simulink model "EvBoltCalib_Lat_v1_comb"  (R2022b)
settings: configuration reference "ConfigSetDesktopFixedStep" (kept outside this file)
PreLoadFcn:
  | VSS_BICYCLE=Simulink.Variant('Dual=0');
  | VSS_DUAL=Simulink.Variant('Dual=1');
  | Dual=1;
undefined symbols (not defined in the file or in its folder): BattChargeLimitMaxPwr, BattChargeLimitSocBpts, BattChargeLimitTbl, BattChrgCapcty, BattDischargeLimitSocBpts, BattDischargeLimitTbl, BattDischargeMaxPwr, BattNumCellsParallel, BattNumCellsSeries, BattOpenVoltCapBpts, BattOpenVoltTbl, BattResistSocBpts, BattResistTbl, BattResistTempBpts, BrakeMaxPrs, BrakeMaxTrq, ChassisDistCg2FrontAxle, ChassisDistCg2RearAxle, ChassisVehMass, DiffRatio, EnvGravCnst, EnvPrs, EnvTemp, ExpRefStructs, FuelSpecificGrav, h, InitStates, MtrEffSpdBpts, MtrEffTbl, MtrEffTrqBpts, MtrPwrMax, MtrTrqMax, SupvsryCtrlRegenBrkCutOffTbl, SupvsryCtrlRegenSpdBpts, TestScnrioCycleNum, VEH
libraries: vehdynlibtire x8, vehdynlibsuspension x7, autolibshared x6, simulink x6, autolibutils x5, VsrLibWheel x4, vehdynlibtirecommon x3, sharedtransform x3, autolibbatterycommon x2, autolibpowerinfoutils x2, autolibsharedcoupling x2, LibPtSupervisoryCtrl x2
(part 2 of 9)

== system EvBoltCalib_Lat_v1_comb/Driver/Vehicle Dynamics Blockset Complete Driver/Complete Driver ==
  TestScnrio : Inport
  Env : Inport  Port=2
  Veh : Inport  Port=3
  Bus Selector1 : BusSelector  OutputSignals=VehRefSpdLookAhead,LatRef.LatCoGDisp,GradeLookAhead
  Bus Selector2 : BusSelector  OutputSignals=Chassis.xdot,Chassis.Y,Chassis.ydot,Chassis.psi,Chassis.r
  Constant : Constant
  Constant1 : Constant
  Constant2 : Constant  Value=0
  Dead Zone : DeadZone  LowerValue=-1e-2  UpperValue=1e-2  ZeroCross=off
  Dead Zone1 : DeadZone  ZeroCross=off
  Gain : Gain  Gain=20*pi/180*18
  Predictive Driver : vehdynlibdriver/Predictive Driver  extAccelOvr=off  extDecelOvr=off  extAccelHld=off  extDecelHld=off  extAccelZero=off  extDecelZero=off  extSteerOvr=off  extSteerHld=off  extSteerZero=off  cntrlType=PI  cntrlTypeLat=Predictive  shftType=None  coordMode=SAE J670 (Z-down)  refType=Reference pose  velUnits=m/s  angUnits=rad  gearOut=off  steerOut=off  Kp=10  Ki=5  Kff=.1  Kg=0  VehVelVec=[0 100]  KffVec=[.1 .1]  KpVec=[5 5]  KiVec=[5 5]  KgVec=[0 0]  vnom=5  Kaw=1  tauerr=.01  tau=0.03  L=1  Kpt=20000  aR=200  bR=2.5  cR=.5  g=9.81  vecPose=off  dynamMode=off  PositionGainF=2.5  PositionGainR=2.5  YawRateGain=.2  DelayGain=.2  enableDrift=off  BetaRef=20*pi/180  KpBeta=1  KpDrift=2  KdDrift=1  KpPsi=6  KOmega=30  tOmega=1  a=ChassisDistCg2FrontAxle  b=ChassisDistCg2RearAxle  m=ChassisVehMass  Cy_f=5000  Cy_r=7000  I=2066  Ksteer=18  theta=40*pi/180  Idl=3  Re=.3  lambda_mu=1  GearInit=0  tShift=.1  pdlVec=[0.1 0.4 0.5 0.9]  upShftTbl=[-1 12.9375 26.4375 39.9375 51.18749999999999 62.4375 72.84375 83.25;-1 16.3125 29.8125 43.3125 54.5624 65.8125 76.78125 87.75;-1 19.6875 33.1875 46.68749999999999 57.9375 69.1875 80.71875 92.25;-1 33 52.5 77.25 100.5 138.75 161.875 185]  dwnShftTbl=[-1 12.9375 26.4375 39.9375 51.18749999999999 62.4375 72.84375 83.25;-1 16.3125 29.8125 43.3125 54.5624 65.8125 76.78125 87.75;-1 19.6875 33.1875 46.68749999999999 57.9375 69.1875 80.71875 92.25;-1 33 52.5 77.25 100.5 138.75 161.875 185]  tClutch=.5  tRev=.5  tPark=120  UpGearVec="[0  1  2  3  4  5  6  7]"  DownGearVec="[1  2  3  4  5  6  7  8]"  aMode=2
  Terminator : Terminator
  Terminator6 : Terminator
  AccelCmd : Outport
  DecelCmd : Outport  Port=2
  GearCmd : Outport  Port=3
  CltchCmd : Outport  Port=4
  IgSw : Outport  Port=5
  SteerCmd : Outport  Port=6
  wires:
  Constant/1 -> IgSw/1
  Constant1/1 -> GearCmd/1
  Env/1 -> Terminator/1
  Constant2/1 -> CltchCmd/1
  Veh/1 -> Bus Selector2/1
  Predictive Driver/3 -> AccelCmd/1
  Predictive Driver/4 -> DecelCmd/1
  Predictive Driver/2 -> Dead Zone/1
  Predictive Driver/1 -> Terminator6/1
  Dead Zone/1 -> Gain/1
  Gain/1 -> SteerCmd/1
  TestScnrio/1 -> Bus Selector1/1
  Bus Selector1/1 -> Predictive Driver/1  "<VehRefSpdLookAhead>"
  Bus Selector1/2 -> Predictive Driver/2  "<LatCoGDisp>"
  Bus Selector1/3 -> Predictive Driver/3  "<GradeLookAhead>"
  Bus Selector2/1 -> Dead Zone1/1  "<xdot>"
  Dead Zone1/1 -> Predictive Driver/4
  Bus Selector2/2 -> Predictive Driver/5  "<Y>"
  Bus Selector2/3 -> Predictive Driver/6  "<ydot>"
  Bus Selector2/4 -> Predictive Driver/7  "<psi>"
  Bus Selector2/5 -> Predictive Driver/8  "<r>"

== system EvBoltCalib_Lat_v1_comb/Driver/Vehicle Dynamics Blockset Complete Driver/Subsystem3 ==
  AccelCmd : Inport
  DecelCmd : Inport  Port=2
  GearCmd : Inport  Port=3
  CltchCmd : Inport  Port=4
  IgSw : Inport  Port=5
  SteeringCmd : Inport  Port=6
  Bus Creator : BusCreator  Inputs=6
  TransPlant : Outport
  wires:
  AccelCmd/1 -> Bus Creator/1  "AccelCmd"
  DecelCmd/1 -> Bus Creator/2  "DecelCmd"
  Bus Creator/1 -> TransPlant/1  "Driver"
  GearCmd/1 -> Bus Creator/3  "GearCmd"
  CltchCmd/1 -> Bus Creator/4  "CltchCmd"
  IgSw/1 -> Bus Creator/5  "IgSw"
  SteeringCmd/1 -> Bus Creator/6  "SteeringCmd"

== system EvBoltCalib_Lat_v1_comb/Driver/Vehicle Dynamics Blockset Longitudinal Driver /Longitudinal Driver ==
  VehRefSpd : Inport
  VehRefSpdLookAhead : Inport  Port=2
  VehDistLookAhead : Inport  Port=3
  TimeLookAhead : Inport  Port=4
  VehSpd : Inport  Port=5
  VehDist : Inport  Port=6
  RoadGrade : Inport  Port=7
  GradeLookAhead : Inport  Port=8
  Add : Sum  Inputs=+-
  Constant : Constant
  Constant1 : Constant
  Constant2 : Constant  Value=0
  Longitudinal Driver : autolibshared/Longitudinal Driver  extAccelOvr=off  extDecelOvr=off  extAccelHld=off  extDecelHld=off  extAccelZero=off  extDecelZero=off  cntrlType=PI  shftType=None  velUnits=m/s  gearOut=off  Kp=5  Ki=1  Kff=.1  Kg=0  VehVelVec=[0 100]  KffVec=[.1 .1]  KpVec=[10 10]  KiVec=[5 5]  KgVec=[0 0]  m=ChassisVehMass  Kpt=3000  tau=0.5  L=3  aR=200  bR=2.5  cR=.5  g=9.81  vnom=5  Kaw=1  tauerr=.01  tauPt=2  GearInit=0  tShift=.1  pdlVec=[0.1 0.4 0.5 0.9]  upShftTbl=[-1 12.9375 26.4375 39.9375 51.18749999999999 62.4375 72.84375 83.25;-1 16.3125 29.8125 43.3125 54.5624 65.8125 76.78125 87.75;-1 19.6875 33.1875 46.68749999999999 57.9375 69.1875 80.71875 92.25;-1 33 52.5 77.25 100.5 138.75 161.875 185]  dwnShftTbl=[1 9.5625 23.0625 36.5625 47.8125 59.0625 68.90625 78.75;1 12.9375 26.4375 39.9375 51.18749999999999 62.4375 72.84375 83.25;1 16.3125 29.8125 43.3125 54.562499 65.8125 76.78125 87.75;1 19.6875 33.1875 46.68749999999999 57.9375 69.1875 80.71875 92.25]  tClutch=.5  tRev=.5  tPark=120  aMode=2  UpGearVec="[0  1  2  3  4  5  6  7]"  DownGearVec="[1  2  3  4  5  6  7  8]"
  Scope : Scope
  Terminator{,1..5} (6 alike) : Terminator
  AccelCmd : Outport
  DecelCmd : Outport  Port=2
  GearCmd : Outport  Port=3
  CltchCmd : Outport  Port=4
  IgSw : Outport  Port=5
  wires:
  VehRefSpd/1 -> Longitudinal Driver/1
  RoadGrade/1 -> Longitudinal Driver/3
  VehSpd/1 -> Longitudinal Driver/2
  Constant/1 -> IgSw/1
  Constant1/1 -> GearCmd/1
  GradeLookAhead/1 -> Terminator4/1
  VehRefSpdLookAhead/1 -> Terminator/1
  TimeLookAhead/1 -> Terminator2/1
  Longitudinal Driver/2 -> AccelCmd/1
  Longitudinal Driver/3 -> DecelCmd/1
  Constant2/1 -> CltchCmd/1
  VehDistLookAhead/1 -> Add/1, Terminator1/1
  VehDist/1 -> Add/2, Terminator3/1
  Longitudinal Driver/1 -> Terminator5/1
  Add/1 -> Scope/1

== system EvBoltCalib_Lat_v1_comb/Driver/Vehicle Dynamics Blockset Longitudinal Driver /Subsystem1 ==
  AccelCmd : Inport
  DecelCmd : Inport  Port=2
  GearCmd : Inport  Port=3
  CltchCmd : Inport  Port=4
  IgSw : Inport  Port=5
  SteeringCmd : Inport  Port=6
  Bus Creator : BusCreator  Inputs=6
  TransPlant : Outport
  wires:
  AccelCmd/1 -> Bus Creator/1  "AccelCmd"
  DecelCmd/1 -> Bus Creator/2  "DecelCmd"
  Bus Creator/1 -> TransPlant/1  "Driver"
  GearCmd/1 -> Bus Creator/3  "GearCmd"
  CltchCmd/1 -> Bus Creator/4  "CltchCmd"
  IgSw/1 -> Bus Creator/5  "IgSw"
  SteeringCmd/1 -> Bus Creator/6  "SteeringCmd"

== system EvBoltCalib_Lat_v1_comb/Driver/Vehicle Dynamics Blockset Longitudinal Driver /Subsystem2 ==
  TestScnrio : Inport
  Env : Inport  Port=2
  Veh : Inport  Port=3
  Bus Selector : BusSelector  OutputSignals=VehRefSpd,VehRefSpdLookAhead,VehDistLookAhead,VehDist,GradeLookAhead,TimeLookAhead
  Bus Selector1 : BusSelector  OutputSignals=RoadGrade
  Bus Selector2 : BusSelector  OutputSignals=Chassis.VehSpd
  VehRefSpd : Outport
  VehRefSpdLookAhead : Outport  Port=2
  VehDistLookAhead : Outport  Port=3
  TimeLookAhead : Outport  Port=4
  VehSpd : Outport  Port=5
  VehDist : Outport  Port=6
  RoadGrade : Outport  Port=7
  GradeLookAhead : Outport  Port=8
  wires:
  TestScnrio/1 -> Bus Selector/1
  Env/1 -> Bus Selector1/1
  Bus Selector1/1 -> RoadGrade/1  "<RoadGrade>"
  Veh/1 -> Bus Selector2/1
  Bus Selector2/1 -> VehSpd/1  "<VehSpd>"
  Bus Selector/1 -> VehRefSpd/1  "<VehRefSpd>"
  Bus Selector/2 -> VehRefSpdLookAhead/1  "<VehRefSpdLookAhead>"
  Bus Selector/3 -> VehDistLookAhead/1  "<VehDistLookAhead>"
  Bus Selector/4 -> VehDist/1  "<VehDist>"
  Bus Selector/5 -> GradeLookAhead/1  "<GradeLookAhead>"
  Bus Selector/6 -> TimeLookAhead/1  "<TimeLookAhead>"

== system EvBoltCalib_Lat_v1_comb/Environment/Ground Feedback/3D Engine ==
  Friction : Inport
  Ground Z Level : Inport  Port=2
  Bus Creator : BusCreator  Inputs=4
  Bus Creator2 : BusCreator  Inputs=4
  Bus Creator3 : BusCreator  Inputs=2
  Bus Selector : BusSelector  OutputSignals=HitLoc
  Data Type Conversion : DataTypeConversion  SaturateOnIntegerOverflow=off  RndMeth=Floor
  Demux : Demux
  Demux1 : Demux
  Passenger Vehicle Ray Trace Set : sim3dlib/Vehicle Terrain Sensor  Priority=1  ActorTag=SimulinkVehicle1  VehExtEn=Constant  TireRadiiExt=Constant  VehCntrLngthVal=0  TireRadiiVal=0  VehRayLngth=10  LfRayLngth=20  RfRayLngth=20  LrRayLngth=20  RrRayLngth=20  VehRayOffset=0  LfRayOffset=-1  RfRayOffset=-1  LrRayOffset=-1  RrRayOffset=-1  VehEn=on  LfEn=on  RfEn=on  LrEn=on  RrEn=on  DbgEn=off  Ts=.03  aMode=aMode
  Rate Transition : RateTransition
  Reshape10 : Reshape  OutputDimensionality=Row vector (2-D)
  Selector1 : Selector  InputPortWidth=5  IndexOptions=Index vector (dialog)  Indices=[2:5]  OutputSizes=1
  Signal Specification : SignalSpecification  Unit=m
  Signal Specification1 : SignalSpecification  Unit=1
  Terminator : Terminator
  Terminator1 : Terminator
  Terminator2 : Terminator
  Zend Select : Selector  NumberOfDimensions=2  InputPortWidth=3  IndexOptions=Select all,Index vector (dialog)  Indices=[1 3],3  OutputSizes=1,1
  Ground : Outport  VectorParamsAs1DForOutWhenUnconnected=off
  wires:
  Selector1/1 -> Rate Transition/1
  Zend Select/1 -> Reshape10/1
  Bus Selector/1 -> Zend Select/1  "<HitLoc>"
  Passenger Vehicle Ray Trace Set/2 -> Terminator1/1
  Passenger Vehicle Ray Trace Set/3 -> Terminator2/1
  Reshape10/1 -> Selector1/1
  Passenger Vehicle Ray Trace Set/1 -> Bus Selector/1
  Rate Transition/1 -> Data Type Conversion/1
  Demux/2 -> Bus Creator/2  "G_FR_z"
  Demux/1 -> Bus Creator/1  "G_FL_z"
  Demux/4 -> Bus Creator/4  "G_RR_z"
  Demux/3 -> Bus Creator/3  "G_RL_z"
  Signal Specification/1 -> Demux/1
  Signal Specification1/1 -> Demux1/1
  Demux1/1 -> Bus Creator2/1  "mu_FL"
  Bus Creator/1 -> Bus Creator3/1  "z"
  Demux1/3 -> Bus Creator2/3  "mu_RL"
  Demux1/4 -> Bus Creator2/4  "mu_RR"
  Demux1/2 -> Bus Creator2/2  "mu_FR"
  Bus Creator2/1 -> Bus Creator3/2  "mu"
  Bus Creator3/1 -> Ground/1
  Friction/1 -> Signal Specification1/1
  Data Type Conversion/1 -> Signal Specification/1
  Ground Z Level/1 -> Terminator/1

== system EvBoltCalib_Lat_v1_comb/Environment/Ground Feedback/Constant ==
  Friction : Inport
  Ground Z Level : Inport  Port=2
  Bus Creator : BusCreator  Inputs=4
  Bus Creator2 : BusCreator  Inputs=4
  Bus Creator3 : BusCreator  Inputs=2
  Demux : Demux
  Demux1 : Demux
  Signal Specification : SignalSpecification  Unit=m
  Signal Specification1 : SignalSpecification  Unit=1
  Ground : Outport  VectorParamsAs1DForOutWhenUnconnected=off
  wires:
  Ground Z Level/1 -> Signal Specification/1
  Signal Specification/1 -> Demux/1
  Demux/4 -> Bus Creator/4  "G_RR_z"
  Demux/1 -> Bus Creator/1  "G_FL_z"
  Demux/3 -> Bus Creator/3  "G_RL_z"
  Demux/2 -> Bus Creator/2  "G_FR_z"
  Bus Creator/1 -> Bus Creator3/1  "z"
  Demux1/3 -> Bus Creator2/3  "mu_RL"
  Demux1/4 -> Bus Creator2/4  "mu_RR"
  Demux1/1 -> Bus Creator2/1  "mu_FL"
  Demux1/2 -> Bus Creator2/2  "mu_FR"
  Bus Creator2/1 -> Bus Creator3/2  "mu"
  Friction/1 -> Signal Specification1/1
  Signal Specification1/1 -> Demux1/1
  Bus Creator3/1 -> Ground/1

== system EvBoltCalib_Lat_v1_comb/Test Scenario/Drive Cycle Source/Subsystem1 ==
  LatCoGDispRef : Inport  Unit=m
  SteeringRef : Inport  Port=2  Unit=rad
  Bus Creator : BusCreator  Inputs=2
  LatRef : Outport
  wires:
  LatCoGDispRef/1 -> Bus Creator/1  "LatCoGDisp"
  Bus Creator/1 -> LatRef/1  "LatRef"
  SteeringRef/1 -> Bus Creator/2  "Steering"

== system EvBoltCalib_Lat_v1_comb/Vehicle/Battery/Battery ==
  note: Thermal model is needed to estimated battery temperature. Ambient temperture is assumed.
  Bus Creator1 : BusCreator  Inputs=1
  Bus Selector : BusSelector  OutputSignals=BattSoc
  Bus Selector2 : BusSelector  OutputSignals=Curr
  Constant : Constant  Value=EnvTemp
  Lithium Ion Battery Pack1 : Subsystem  AncestorBlock=autolibdatasheetbattery/Datasheet Battery  mask(Datasheet Battery){CapacityCtrl=Parameter, OutputVlt=Unfiltered, BattChargeMax=BattChrgCapcty, Em=BattOpenVoltTbl, CapLUTBp=BattOpenVoltCapBpts, RInt=BattResistTbl, BattTempBp=BattResistTempBpts, CapSOCBp=BattResistSocBpts, Ns=BattNumCellsSeries, Np=BattNumCellsParallel, BattCapInit=InitStates(TestScnrioCycleNum).BattSoc*BattChrgCapcty, Tc=1/1000, Vinit=3.75*72, RefBlkName='autolibdatasheetbattery/Datasheet Battery'}
      mask prompts: CapacityCtrl "autoblks:autoblkDatasheetBattery:blkPrm_CapacityCtrl"; OutputVlt "autoblks:autoblkDatasheetBattery:blkPrm_OutputVlt"; BattChargeMax "autoblks:autoblkDatasheetBattery:blkPrm_BattChargeMax"; Em "autoblks:autoblkDatasheetBattery:blkPrm_Em"; CapLUTBp "autoblks:autoblkDatasheetBattery:blkPrm_CapLUTBp"; RInt "autoblks:autoblkDatasheetBattery:blkPrm_RInt"; BattTempBp "autoblks:autoblkDatasheetBattery:blkPrm_BattTempBp"; CapSOCBp "autoblks:autoblkDatasheetBattery:blkPrm_CapSOCBp"; Ns "autoblks:autoblkDatasheetBattery:blkPrm_Ns"; Np "autoblks:autoblkDatasheetBattery:blkPrm_Np"; BattCapInit "autoblks:autoblkDatasheetBattery:blkPrm_BattCapInit"; Tc "autoblks:autoblkDatasheetBattery:blkPrm_Tc"; Vinit "autoblks:autoblkDatasheetBattery:blkPrm_Vinit"
      mask help: autoblks:autoblkDatasheetBattery:blkDesc
      mask init:
      | autoicon('autolibdatasheetbattery',gcb,'Initialization');
      settings: LibrarySourceBlock=autolibdatasheetbattery/Datasheet Battery
      mask Help: eval('autoblkshelp(''pbbatterydatasheet'')');
      mask TypeOptions CapacityCtrl: autoblks:autoblkDatasheetBattery:blkCmb_CapacityCtrlExternalInput | autoblks:autoblkDatasheetBattery:blkCmb_CapacityCtrlParameter
      mask TypeOptions OutputVlt: autoblks:autoblkDatasheetBattery:blkCmb_OutputVltFiltered | autoblks:autoblkDatasheetBattery:blkCmb_OutputVltUnfiltered
      mask DialogControl Container3 Prompt: autoblks:autoblkDatasheetBattery:blkDlg_Container3
      mask DialogControl CapacityCtrl Prompt: Initial battery capacity:
      mask DialogControl OutputVlt Prompt: Output battery voltage:
      mask DialogControl ParameterGroupVar Prompt: autoblks:autoblkDatasheetBattery:blkDlg_ParameterGroupVar
      mask DialogControl BattChargeMax Prompt: Rated capacity at nominal temperature, BattChargeMax [Ah]:
      mask DialogControl Em Prompt: Open circuit voltage table data, Em [V]:
      mask DialogControl CapLUTBp Prompt: Open circuit voltage breakpoints 1, CapLUTBp []:
      mask DialogControl RInt Prompt: Internal resistance table data, RInt [Ohms]:
      mask DialogControl BattTempBp Prompt: Battery temperature breakpoints 1, BattTempBp [K]:
      mask DialogControl CapSOCBp Prompt: Battery capacity breakpoints 2, CapSOCBp []:
      mask DialogControl Ns Prompt: Number of cells in series, Ns []:
      mask DialogControl Np Prompt: Number of cells in parallel, Np []:
      mask DialogControl BattCapInit Prompt: Initial battery capacity, BattCapInit [Ah]:
      mask DialogControl Tc Prompt: Output battery voltage time constant, Tc [s]:
      mask DialogControl Vinit Prompt: Output battery voltage initial value, Vinit [V]:
      mask Display:
      | IconInfo = autoicon('autolibdatasheetbattery', gcb, 'DrawCommands');
      | 
      | image(IconInfo.image, IconInfo.position);
      | 
      | for i = 1:numel(IconInfo.lconn)
      |     port_label('lconn', i, IconInfo.lconn{i})
      | end
      | 
      | for j = 1:numel(IconInfo.rconn)
      |     port_label('rconn', j, IconInfo.rconn{j})
      | end
      | 
      | for k = 1:numel(IconInfo.input)
      |     port_label('input', k, IconInfo.input{k})
      | end
      | 
      | for m = 1:numel(IconInfo.output)
      |     port_label('output', m, IconInfo.output{m})
      | end
  Two-Way Connection1 : TwoWayConnection
  Batt : PMIOPort  Side=Right
  BattSoc : Outport
  BattCurr : Outport  Port=2  Unit=A
  BattVolt : Outport  Port=3  Unit=V
  wires:
  Bus Selector2/1 -> Lithium Ion Battery Pack1/1(BattCurr), BattCurr/1  "<Curr>"
  Lithium Ion Battery Pack1/2(BattVolt) -> BattVolt/1, Bus Creator1/1  "Volt"
  Bus Creator1/1 -> Two-Way Connection1/1
  Constant/1 -> Lithium Ion Battery Pack1/2(BattTemp)
  Bus Selector/1 -> BattSoc/1  "<BattSoc>"
  Lithium Ion Battery Pack1/1(Info) -> Bus Selector/1
  Two-Way Connection1/1 -> Bus Selector2/1
  connections:
  Batt/RConn1 -- Two-Way Connection1/RConn1

== system EvBoltCalib_Lat_v1_comb/Vehicle/Battery/Subsystem1 ==
  BattSoc : Inport
  BattCurr : Inport  Port=2
  BattVolt : Inport  Port=3
  Bus Creator : BusCreator  Inputs=3
  Batt : Outport
  wires:
  BattSoc/1 -> Bus Creator/1  "BattSoc"
  BattCurr/1 -> Bus Creator/2  "BattCurr"
  Bus Creator/1 -> Batt/1  "Batt"
  BattVolt/1 -> Bus Creator/3  "BattVolt"

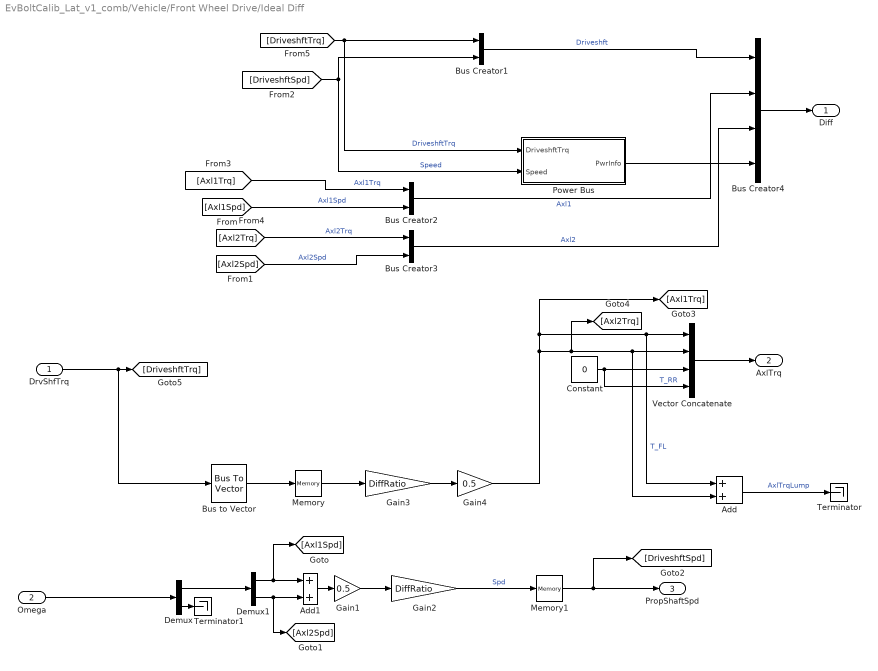
== system EvBoltCalib_Lat_v1_comb/Vehicle/Front Wheel Drive/Ideal Diff ==
  DrvShfTrq : Inport
  Omega : Inport  Port=2
  Add : Sum
  Add1 : Sum
  Bus Creator1 : BusCreator  Inputs=2
  Bus Creator2 : BusCreator  Inputs=2
  Bus Creator3 : BusCreator  Inputs=2
  Bus Creator4 : BusCreator  Inputs=4
  Bus to Vector : BusToVector
  Constant : Constant  Value=0
  Demux : Demux  Outputs=[2,2]
  Demux1 : Demux  Outputs=2
  Gain1 : Gain  Gain=0.5
  Gain2 : Gain  Gain=DiffRatio
  Gain3 : Gain  Gain=DiffRatio
  Gain4 : Gain  Gain=0.5
  Memory : Memory
  Memory1 : Memory
  Power Bus : Subsystem
  Terminator : Terminator
  Terminator1 : Terminator
  Vector Concatenate : Concatenate  NumInputs=4
  Diff : Outport  VectorParamsAs1DForOutWhenUnconnected=off
  AxlTrq : Outport  Port=2  VectorParamsAs1DForOutWhenUnconnected=off
  PropShaftSpd : Outport  Port=3  VectorParamsAs1DForOutWhenUnconnected=off
  wires:
  Demux1/2 -> [Axl2Spd], Add1/2
  Vector Concatenate/1 -> AxlTrq/1
  Gain4/1 -> [Axl1Trq], Add/1, Vector Concatenate/1, [Axl2Trq], Add/2, Vector Concatenate/2  "T_FL"
  DrvShfTrq/1 -> [DriveshftTrq], Bus to Vector/1
  [DriveshftTrq] -> Power Bus/1(DriveshftTrq), Bus Creator1/1  "DriveshftTrq"
  [Axl1Spd] -> Bus Creator2/2  "Axl1Spd"
  Demux/1 -> Demux1/1
  Add1/1 -> Gain1/1
  Bus Creator4/1 -> Diff/1
  Add/1 -> Terminator/1  "AxlTrqLump"
  [Axl2Trq] -> Bus Creator3/1  "Axl2Trq"
  Omega/1 -> Demux/1
  Memory/1 -> Gain3/1
  Bus to Vector/1 -> Memory/1
  Bus Creator3/1 -> Bus Creator4/3  "Axl2"
  Bus Creator2/1 -> Bus Creator4/2  "Axl1"
  Bus Creator1/1 -> Bus Creator4/1  "Driveshft"
  [DriveshftSpd] -> Bus Creator1/2, Power Bus/2(Speed)  "Speed"
  Gain2/1 -> Memory1/1  "Spd"
  Constant/1 -> Vector Concatenate/4, Vector Concatenate/3  "T_RR"
  Demux1/1 -> [Axl1Spd], Add1/1
  Memory1/1 -> PropShaftSpd/1, [DriveshftSpd]
  Gain3/1 -> Gain4/1
  [Axl1Trq] -> Bus Creator2/1  "Axl1Trq"
  Power Bus/1(PwrInfo) -> Bus Creator4/4
  Gain1/1 -> Gain2/1
  [Axl2Spd] -> Bus Creator3/2  "Axl2Spd"
  Demux/2 -> Terminator1/1

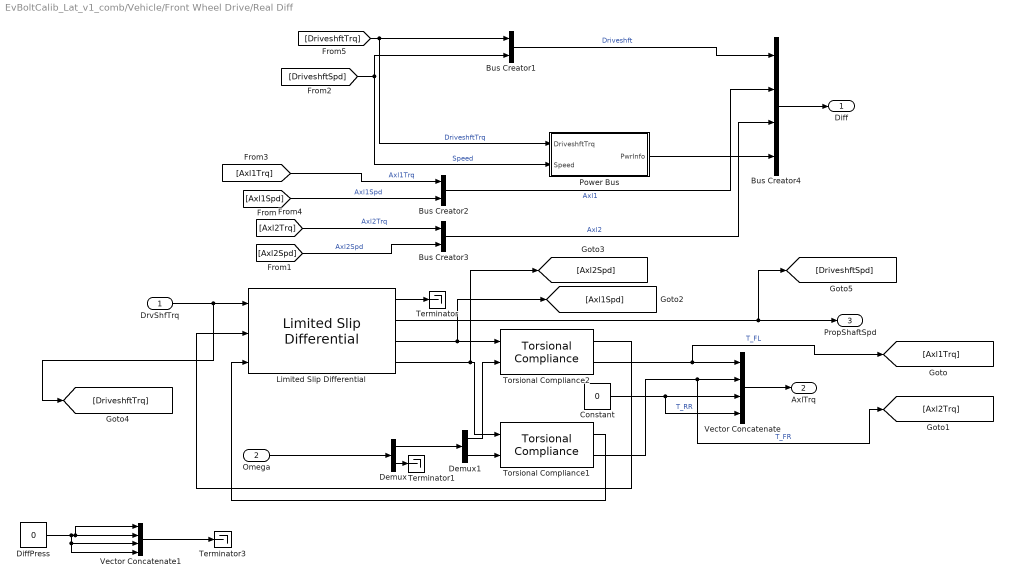
== system EvBoltCalib_Lat_v1_comb/Vehicle/Front Wheel Drive/Real Diff ==
  DrvShfTrq : Inport
  Omega : Inport  Port=2
  Bus Creator1 : BusCreator  Inputs=2
  Bus Creator2 : BusCreator  Inputs=2
  Bus Creator3 : BusCreator  Inputs=2
  Bus Creator4 : BusCreator  Inputs=4
  Constant : Constant  Value=0
  Demux : Demux  Outputs=[2,2]
  Demux1 : Demux  Outputs=2
  DiffPress : Constant  Value=0
  Limited Slip Differential : autolibshareddiff/Limited Slip Differential  DiffEffModelPopup=Constant  InterpMethod=Linear point-slope  extTamb=off  shaftSwitchMask=To the left of center-line  Ndiff=7.05  Jd=0.025  bd=1e-3  Jw1=0.01  bw1=1e-3  Jw2=0.01  bw2=1e-3  omegaw1o=0  omegaw2o=0  eta=0.98  eta_tbl=reshape([0.64 0.76 0.8 0.81 0.83 0.84 0.84 0.56 0.73 0.78 0.8 0.83 0.84 0.84 0.54 0.71 0.77 0.8 0.82 0.84 0.84 0.53 0.71 0.77 0.8 0.83 0.84 0.84 0.51 0.71 0.77 0.8 0.83 0.84 0.85 0.52 0.7 0.77 0.8 0.83 0.84 0.85 0.51 0.71 0.76 0.79 0.83 0.84 0.85 0.5 0.69 0.76 0.79 0.82 0.84 0.85 0.45 0.68 0.75 0.78 0.82 0.84 0.85 0.43 0.67 0.74 0.78 0.81 0.83 0.84 0.38 0.63 0.71 0.75 0.8 0.82 0.83 0.81 0.86 0.88 0.89 0.89 0.89 0.9 0.77 0.85 0.87 0.88 0.89 0.9 0.9 0.72 0.82 0.86 0.87 0.88 0.89 0.9 0.68 0.8 0.84 0.86 0.88 0.89 0.89 0.67 0.8 0.84 0.86 0.88 0.89 0.9 0.67 0.8 0.84 0.86 0.88 0.89 0.9 0.65 0.8 0.84 0.86 0.88 0.89 0.9 0.64 0.79 0.83 0.86 0.88 0.89 0.9 0.63 0.78 0.83 0.86 0.88 0.89 0.9 0.59 0.76 0.82 0.85 0.87 0.89 0.9 0.53 0.73 0.8 0.83 0.86 0.88 0.89], 7, 11, 2)  Trq_bpts=[25, 50, 75, 100, 150, 200, 250]  omega_bpts=[52.4 78.5 105 131 157 183 209 262 314 419 524]  Temp_bpts=[290 358]  Tamb=297.15  couplingType=Pre-loaded ideal clutch  Ndisks=8  Reff=.08  Fc=1000  muc=[.16 0.13 0.115 0.11 0.105 0.1025 0.10125 .10125]  dw=[0 10 20 40 60 80 100 1000]  Tdw=[-100, -90, -50, -5, 0, 5, 50, 90, 100]  dwT=[-200, -175, -100, - 50, 0, 50, 100, 175, 200]  TTin=[-200 -175 -100 - 50 0 50 100 175 200]  Tin=[-200 -175 -100 - 50 0 50 100 175 200]  tauC=.04  IdealInterpMethod=Linear point-slope  IdealExtrapMethod=Linear  TdwInterpMethod=Flat  TdwExtrapMethod=Clip  TTinInterpMethod=Flat  TTinExtrapMethod=Clip  maxAbsSpd=5e3  aMode=2
  Power Bus : Subsystem
  Terminator : Terminator
  Terminator1 : Terminator
  Terminator3 : Terminator
  Torsional Compliance1 : autolibsharedcoupling/Torsional Compliance  port_config=Simulink  extInfo=off  k=10000  b=400  theta_o=0  domega_o=0  omega_c=300  blkID=0  aMode=2
  Torsional Compliance2 : autolibsharedcoupling/Torsional Compliance  port_config=Simulink  extInfo=off  k=10000  b=400  theta_o=0  domega_o=0  omega_c=300  blkID=0  aMode=2
  Vector Concatenate : Concatenate  NumInputs=4
  Vector Concatenate1 : Concatenate  NumInputs=4
  Diff : Outport  VectorParamsAs1DForOutWhenUnconnected=off
  AxlTrq : Outport  Port=2  VectorParamsAs1DForOutWhenUnconnected=off
  PropShaftSpd : Outport  Port=3  VectorParamsAs1DForOutWhenUnconnected=off
  wires:
  Limited Slip Differential/3 -> [Axl1Spd], Torsional Compliance2/1
  Demux1/1 -> Torsional Compliance2/2
  Limited Slip Differential/1 -> Terminator/1
  DrvShfTrq/1 -> [DriveshftTrq], Limited Slip Differential/1
  Limited Slip Differential/4 -> [Axl2Spd], Torsional Compliance1/1
  Demux1/2 -> Torsional Compliance1/2
  Demux/1 -> Demux1/1
  Torsional Compliance1/1 -> Limited Slip Differential/3
  Torsional Compliance2/1 -> Limited Slip Differential/2
  Demux/2 -> Terminator1/1
  Constant/1 -> Vector Concatenate/4, Vector Concatenate/3  "T_RR"
  Torsional Compliance1/2 -> [Axl2Trq], Vector Concatenate/2  "T_FR"
  Torsional Compliance2/2 -> [Axl1Trq], Vector Concatenate/1  "T_FL"
  Omega/1 -> Demux/1
  Vector Concatenate/1 -> AxlTrq/1
  Vector Concatenate1/1 -> Terminator3/1
  DiffPress/1 -> Vector Concatenate1/4, Vector Concatenate1/3, Vector Concatenate1/1, Vector Concatenate1/2
  [DriveshftTrq] -> Power Bus/1(DriveshftTrq), Bus Creator1/1  "DriveshftTrq"
  [Axl1Spd] -> Bus Creator2/2  "Axl1Spd"
  [Axl2Trq] -> Bus Creator3/1  "Axl2Trq"
  Bus Creator4/1 -> Diff/1
  [Axl2Spd] -> Bus Creator3/2  "Axl2Spd"
  [DriveshftSpd] -> Bus Creator1/2, Power Bus/2(Speed)  "Speed"
  Bus Creator1/1 -> Bus Creator4/1  "Driveshft"
  [Axl1Trq] -> Bus Creator2/1  "Axl1Trq"
  Power Bus/1(PwrInfo) -> Bus Creator4/4
  Bus Creator2/1 -> Bus Creator4/2  "Axl1"
  Bus Creator3/1 -> Bus Creator4/3  "Axl2"
  Limited Slip Differential/2 -> [DriveshftSpd], PropShaftSpd/1

== system EvBoltCalib_Lat_v1_comb/Vehicle/Powertrain Supervisory Controller /Engine Torque Command ==
  AccelCmdIn : Inport
  DecelCmdIn : Inport  Port=2
  DriverGearCmdIn : Inport  Port=3
  VehSpd : Inport  Port=4
  BattSoc : Inport  Port=5
  MtrSpd : Inport  Port=6
  Accel Pedal to Traction Wheel Torque Request1 : Subsystem
  Battery Management System : Subsystem
  Motor Torque Arbitration and Power Management : Subsystem
  Series Regen Braking : Subsystem  InitFcn=%[~]=autosharedicon('autolibutils',gcb,0);  VariantControl=Variant
  MtrTrqCmd : Outport
  AccelCmd : Outport  Port=2
  BrkCmd : Outport  Port=3
  DriverGearCmd : Outport  Port=4
  wires:
  DecelCmdIn/1 -> Series Regen Braking/4("DecelCmd ")  "DecelPdl"
  DriverGearCmdIn/1 -> DriverGearCmd/1
  [AccelPdl] -> Motor Torque Arbitration and Power Management/2(AccelPdl)
  MtrSpd/1 -> [MotSpd], Series Regen Braking/3(MotSpd)  "MotSpd"
  AccelCmdIn/1 -> AccelCmd/1, Accel Pedal to Traction Wheel Torque Request1/1(AccelPdl), [AccelPdl]
  VehSpd/1 -> [VehSpd], Series Regen Braking/2(VehSpd)  "VehSpd"
  BattSoc/1 -> Battery Management System/1(SOC), Series Regen Braking/1(BattSoc)  "SOC"
  Battery Management System/1(BattPwrDischrgLmt) -> Motor Torque Arbitration and Power Management/3(BattPwrDisChrgLmt)  "BattPwrDischrgLmt"
  Series Regen Braking/2(" BrkCmd") -> BrkCmd/1  "BrkCmd"
  Battery Management System/2(BattPwrChrgLmt) -> Motor Torque Arbitration and Power Management/4("BattPwrChrgLmt ")  "BattPwrChrgLmt"
  Series Regen Braking/1(" MotTrqCmdRegen") -> Motor Torque Arbitration and Power Management/6(MotTrqCmdRegen)  "MotTrqCmdRegen"
  [MotSpd] -> Motor Torque Arbitration and Power Management/5(MotSpd)
  Motor Torque Arbitration and Power Management/1(MotTrqCmdFinal) -> MtrTrqCmd/1  "MotTrqCmd"
  [VehSpd] -> Accel Pedal to Traction Wheel Torque Request1/2(MotSpd)
  Accel Pedal to Traction Wheel Torque Request1/1(TrqCmd) -> Motor Torque Arbitration and Power Management/1(MotTrqCmdTrac)

== system EvBoltCalib_Lat_v1_comb/Vehicle/Powertrain Supervisory Controller /Subsystem1 ==
  MtrTrqCmd : Inport
  AccelCmd : Inport  Port=2
  BrkCmd : Inport  Port=3
  DriverGearCmd : Inport  Port=4
  SteeringCmd : Inport  Port=5
  Bus Creator : BusCreator  Inputs=5
  SupvsryCtrl : Outport
  wires:
  MtrTrqCmd/1 -> Bus Creator/1  "MtrTrqCmd"
  Bus Creator/1 -> SupvsryCtrl/1  "SupvsryCtrl"
  AccelCmd/1 -> Bus Creator/2  "AccelCmd"
  BrkCmd/1 -> Bus Creator/3  "BrkCmd"
  DriverGearCmd/1 -> Bus Creator/4  "DriverGearCmd"
  SteeringCmd/1 -> Bus Creator/5  "SteeringCmd"

== system EvBoltCalib_Lat_v1_comb/Vehicle/Powertrain Supervisory Controller /Subsystem4 ==
  Driver : Inport
  Chassis : Inport  Port=2
  Batt : Inport  Port=3
  Mtr : Inport  Port=4
  Bus Selector : BusSelector  OutputSignals=AccelCmd,DecelCmd,GearCmd
  Bus Selector1 : BusSelector  OutputSignals=VehSpd
  Bus Selector2 : BusSelector  OutputSignals=BattSoc
  Bus Selector3 : BusSelector  OutputSignals=MtrSpd
  AccelCmd : Outport  VectorParamsAs1DForOutWhenUnconnected=off
  DecelCmd : Outport  Port=2  VectorParamsAs1DForOutWhenUnconnected=off
  DriverGearCmd : Outport  Port=3  VectorParamsAs1DForOutWhenUnconnected=off
  VehSpd : Outport  Port=4  VectorParamsAs1DForOutWhenUnconnected=off
  BattSoc : Outport  Port=5  VectorParamsAs1DForOutWhenUnconnected=off
  MtrSpd : Outport  Port=6  VectorParamsAs1DForOutWhenUnconnected=off
  wires:
  Driver/1 -> Bus Selector/1
  Bus Selector/1 -> AccelCmd/1  "<AccelCmd>"
  Bus Selector/3 -> DriverGearCmd/1  "<GearCmd>"
  Chassis/1 -> Bus Selector1/1
  Bus Selector1/1 -> VehSpd/1  "<VehSpd>"
  Bus Selector/2 -> DecelCmd/1  "<DecelCmd>"
  Batt/1 -> Bus Selector2/1
  Bus Selector2/1 -> BattSoc/1  "<BattSoc>"
  Mtr/1 -> Bus Selector3/1
  Bus Selector3/1 -> MtrSpd/1  "<MtrSpd>"

== system EvBoltCalib_Lat_v1_comb/Vehicle/Vehicle Dynamics/Vehicle 14DOF ==
  Env : Inport
  SupvsryCtrl : Inport  Port=2
  AxlTrq : Inport  Port=3
  Brake Pressure : Subsystem
  Bus Selector : BusSelector  OutputSignals=SteeringCmd
  Bus Selector1 : BusSelector  OutputSignals=BrkCmd
  Bus Selector2 : BusSelector  OutputSignals=WindVel,GndBus.z,GndBus.mu
  Bus Selector3 : BusSelector  OutputSignals=G_FL_z,G_FR_z,G_RL_z,G_RR_z
  Bus Selector4 : BusSelector  OutputSignals=mu_FL,mu_FR,mu_RL,mu_RR
  Constant : Constant  Value=0
  Steering : Subsystem
  Subsystem4 : Subsystem
  Suspension : Subsystem  Variant=on  VariantControlMode=label  LabelModeActiveChoice=3
      mask Display:
      | switch str2num(get_param(gcb,'ActiveVariant'))
      |     case 1
      |         image('suspdw.png');
      |     case 2
      |         image([imread('suspindmap.png');imread('suspsamap.png')]);
      |     case 3
      |          image([imread('suspmacp.png');imread('suspsacoil.png')]);
      |     case 4
      |          image('suspmacp.png');
      |     case 5
      |          image('suspindmap.png');
      | end
  Vector Concatenate : Concatenate  NumInputs=4
  Vector Concatenate1 : Concatenate  NumInputs=4
  Vector Concatenate2 : Concatenate  NumInputs=4
  Vehicle : Subsystem
      mask Display: image('6dofcar.png');
  Vehicle Routing : Subsystem
  Wheel Routing : Subsystem
  Wheels and Tires : Subsystem
      mask Display: image('wheel3dof.png')
  Whl : Outport
  Chassis : Outport  Port=2
  wires:
  Vehicle Routing/9(GeomXYZdot) -> Subsystem4/9(GeomXYZdot)
  Vehicle Routing/8(GeomXYZ) -> Subsystem4/8(GeomXYZ)
  Vehicle Routing/1(Cgxyzdot) -> Subsystem4/1(Cgxyzdot)
  Vehicle Routing/5(pqr) -> Subsystem4/5(pqr)
  Vehicle Routing/4(angles) -> Subsystem4/4(angles)
  Vehicle Routing/3(CgXYZdot) -> Subsystem4/3(CgXYZdot)
  Vehicle Routing/7(Beta) -> Subsystem4/7(Beta)
  Wheels and Tires/1(Wheels) -> Wheel Routing/2(Wheel), Suspension/3(Wheel)  "Wheels"
  Vehicle Routing/2(CgXYZ) -> Subsystem4/2(CgXYZ)
  Vehicle/1(VehFdbk) -> Suspension/2(Vehicle), Wheel Routing/1(Info), Vehicle Routing/1(Veh)  "Veh"
  Suspension/1(Suspension) -> Vehicle/1(Suspension), Wheels and Tires/1(Suspension)  "Susp"
  Bus Selector2/1 -> Vehicle/2(Wind)  "<WindVel>"
  Steering/1(WhlAng) -> Suspension/1(Steering)
  Bus Selector/1 -> Steering/1(SteeringCmd)  "<SteeringCmd>"
  SupvsryCtrl/1 -> Bus Selector/1, Bus Selector1/1
  Bus Selector1/1 -> Brake Pressure/1(BrkReq)  "<BrkCmd>"
  Env/1 -> Bus Selector2/1
  Vehicle Routing/6(Cgaxyz) -> Subsystem4/6(Cgaxyz)
  Wheel Routing/1(Omega) -> Subsystem4/10(Omega)
  Wheel Routing/3(Alpha) -> Subsystem4/12(Alpha)
  Wheel Routing/4(XWheel) -> Subsystem4/13(XWheel)
  Wheel Routing/2(Kappa) -> Subsystem4/11(Kappa)
  Wheel Routing/5(YWheel) -> Subsystem4/14(YWheel)
  Wheel Routing/6(ZWheel) -> Subsystem4/15(dzWheel)
  Subsystem4/2(Wheels) -> Whl/1
  Subsystem4/1(Chassis) -> Chassis/1
  AxlTrq/1 -> Wheels and Tires/2(Axle Torque)
  Bus Selector2/2 -> Bus Selector3/1  "<z>"
  Bus Selector3/1 -> Vector Concatenate/1  "<G_FL_z>"
  Bus Selector3/2 -> Vector Concatenate/2  "<G_FR_z>"
  Bus Selector3/3 -> Vector Concatenate/3  "<G_RL_z>"
  Bus Selector3/4 -> Vector Concatenate/4  "<G_RR_z>"
  Vector Concatenate/1 -> Wheels and Tires/4(Ground Input)
  Bus Selector4/4 -> Vector Concatenate1/4  "<mu_RR>"
  Bus Selector2/3 -> Bus Selector4/1  "<mu>"
  Bus Selector4/3 -> Vector Concatenate1/3  "<mu_RL>"
  Bus Selector4/2 -> Vector Concatenate1/2  "<mu_FR>"
  Bus Selector4/1 -> Vector Concatenate1/1  "<mu_FL>"
  Vector Concatenate1/1 -> Wheels and Tires/5(Friction)
  Constant/1 -> Vector Concatenate2/4, Vector Concatenate2/3, Vector Concatenate2/2, Vector Concatenate2/1
  Brake Pressure/1(BrakePrs) -> Wheels and Tires/3(Brake Press)

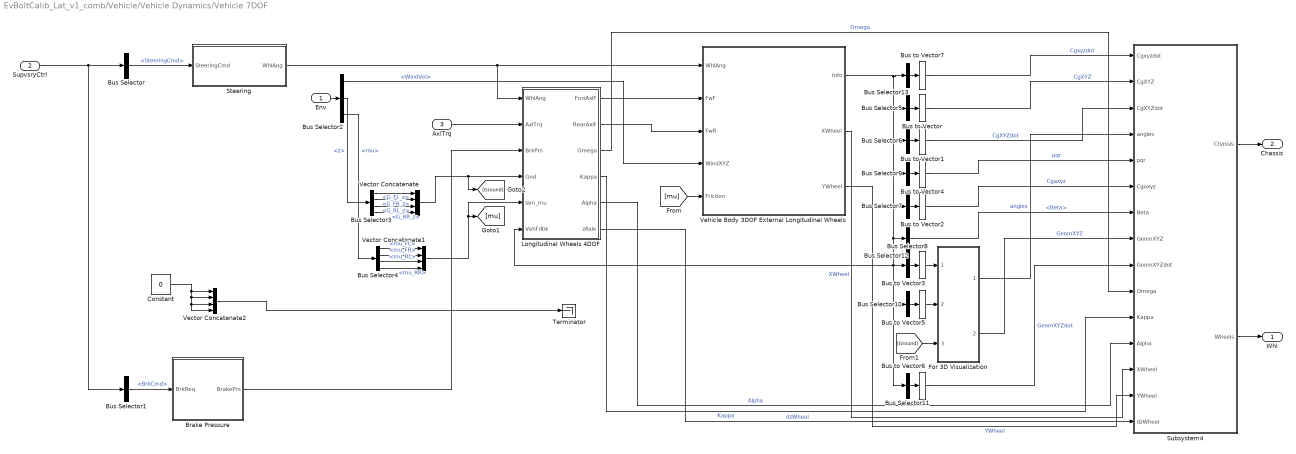
== system EvBoltCalib_Lat_v1_comb/Vehicle/Vehicle Dynamics/Vehicle 7DOF ==
  Env : Inport
  SupvsryCtrl : Inport  Port=2
  AxlTrq : Inport  Port=3
  Brake Pressure : Subsystem
  Bus Selector : BusSelector  OutputSignals=SteeringCmd
  Bus Selector1 : BusSelector  OutputSignals=BrkCmd
  Bus Selector10 : BusSelector  OutputSignals=InertFrm.Geom.Disp.X,InertFrm.Geom.Disp.Y,InertFrm.Geom.Disp.Z  OutputAsBus=on
  Bus Selector11 : BusSelector  OutputSignals=InertFrm.Geom.Vel.Xdot,InertFrm.Geom.Vel.Ydot,InertFrm.Geom.Vel.Zdot  OutputAsBus=on
  Bus Selector12 : BusSelector  OutputSignals=BdyFrm.Geom.Ang.Beta
  Bus Selector13 : BusSelector  OutputSignals=BdyFrm.Cg.Vel.xdot,BdyFrm.Cg.Vel.ydot,BdyFrm.Cg.Vel.zdot  OutputAsBus=on
  Bus Selector2 : BusSelector  OutputSignals=WindVel,GndBus.z,GndBus.mu
  Bus Selector3 : BusSelector  OutputSignals=G_FL_z,G_FR_z,G_RL_z,G_RR_z
  Bus Selector4 : BusSelector  OutputSignals=mu_FL,mu_FR,mu_RL,mu_RR
  Bus Selector5 : BusSelector  OutputSignals=InertFrm.Cg.Disp.X,InertFrm.Cg.Disp.Y,InertFrm.Cg.Disp.Z  OutputAsBus=on
  Bus Selector6 : BusSelector  OutputSignals=InertFrm.Cg.Vel.Xdot,InertFrm.Cg.Vel.Ydot,InertFrm.Cg.Vel.Zdot  OutputAsBus=on
  Bus Selector7 : BusSelector  OutputSignals=BdyFrm.Cg.Acc.ax,BdyFrm.Cg.Acc.ay,BdyFrm.Cg.Acc.az  OutputAsBus=on
  Bus Selector8 : BusSelector  OutputSignals=InertFrm.Cg.Ang.phi,InertFrm.Cg.Ang.theta,InertFrm.Cg.Ang.psi  OutputAsBus=on
  Bus Selector9 : BusSelector  OutputSignals=BdyFrm.Cg.AngVel.p,BdyFrm.Cg.AngVel.q,BdyFrm.Cg.AngVel.r  OutputAsBus=on
  Bus to Vector{,1..7} (8 alike) : BusToVector
  Constant : Constant  Value=0
  For 3D Visualization : MATLAB Function  TreatAsAtomicUnit=on  mask{trackW=1.9, wheelB=ChassisDistCg2FrontAxle+ChassisDistCg2RearAxle}
      mask prompts: trackW "Vehicle track width, trackW [m]:"; wheelB "Vehicle wheelbase, wheelB [m]:"
      mask help: This block converts wheel ground height information into estimates of vehicle pitch, roll angles and vertical height in order to help in the visualization 3DOF based simulations with changes in terrain. Note that the resulting signals are only used as a visualization aid and do not account for the physical affects of the vehicle interacting with variable terrain or changes in orientation.
  Longitudinal Wheels 4DOF : Subsystem  VariantControl=1
      settings: AttributesFormatString=%<wheelMode>
  Steering : Subsystem
  Subsystem4 : Subsystem
  Terminator : Terminator
  Vector Concatenate : Concatenate  NumInputs=4
  Vector Concatenate1 : Concatenate  NumInputs=4
  Vector Concatenate2 : Concatenate  NumInputs=4
  Vehicle Body 3DOF External Longitudinal Wheels : Subsystem  Variant=on  VariantControlMode=label  VariantControl=Variant1  LabelModeActiveChoice=1
      settings: AttributesFormatString=%<trackMode>
  Whl : Outport
  Chassis : Outport  Port=2
  wires:
  Bus Selector2/1 -> Vehicle Body 3DOF External Longitudinal Wheels/4(WindXYZ)  "<WindVel>"
  Bus Selector/1 -> Steering/1(SteeringCmd)  "<SteeringCmd>"
  SupvsryCtrl/1 -> Bus Selector/1, Bus Selector1/1
  Bus Selector1/1 -> Brake Pressure/1(BrkReq)  "<BrkCmd>"
  Env/1 -> Bus Selector2/1
  Subsystem4/2(Wheels) -> Whl/1
  Subsystem4/1(Chassis) -> Chassis/1
  Bus Selector2/2 -> Bus Selector3/1  "<z>"
  Bus Selector3/1 -> Vector Concatenate/1  "<G_FL_z>"
  Bus Selector3/2 -> Vector Concatenate/2  "<G_FR_z>"
  Bus Selector3/3 -> Vector Concatenate/3  "<G_RL_z>"
  Bus Selector3/4 -> Vector Concatenate/4  "<G_RR_z>"
  Bus Selector4/4 -> Vector Concatenate1/4  "<mu_RR>"
  Bus Selector2/3 -> Bus Selector4/1  "<mu>"
  Bus Selector4/3 -> Vector Concatenate1/3  "<mu_RL>"
  Bus Selector4/2 -> Vector Concatenate1/2  "<mu_FR>"
  Bus Selector4/1 -> Vector Concatenate1/1  "<mu_FL>"
  Vector Concatenate2/1 -> Terminator/1
  Constant/1 -> Vector Concatenate2/4, Vector Concatenate2/3, Vector Concatenate2/2, Vector Concatenate2/1
  Bus to Vector2/1 -> Subsystem4/6(Cgaxyz)  "Cgaxyz"
  Bus Selector8/1 -> Bus to Vector3/1
  Bus to Vector5/1 -> For 3D Visualization/2(GemoXYZIn)
  Bus Selector12/1 -> Subsystem4/7(Beta)  "<Beta>"
  Bus Selector5/1 -> Bus to Vector/1
  For 3D Visualization/1(angles) -> Subsystem4/4(angles)  "angles"
  For 3D Visualization/2(GeomXYZ) -> Subsystem4/8(GeomXYZ)  "GeomXYZ"
  Bus to Vector6/1 -> Subsystem4/9(GeomXYZdot)  "GeomXYZdot"
  Bus Selector13/1 -> Bus to Vector7/1
  Bus to Vector7/1 -> Subsystem4/1(Cgxyzdot)  "Cgxyzdot"
  Bus Selector10/1 -> Bus to Vector5/1
  Longitudinal Wheels 4DOF/1(FrntAxlF) -> Vehicle Body 3DOF External Longitudinal Wheels/2("FwF ")
  Bus Selector11/1 -> Bus to Vector6/1
  Bus Selector9/1 -> Bus to Vector4/1
  [mu] -> Vehicle Body 3DOF External Longitudinal Wheels/5(Friction)
  Longitudinal Wheels 4DOF/2(RearAxlF) -> Vehicle Body 3DOF External Longitudinal Wheels/3("FwR ")
  Bus to Vector4/1 -> Subsystem4/5(pqr)  "pqr"
  Vehicle Body 3DOF External Longitudinal Wheels/3(" YWheel") -> Subsystem4/14(YWheel)  "YWheel"
  Vector Concatenate/1 -> Longitudinal Wheels 4DOF/4(Gnd), [Ground]
  Bus to Vector/1 -> Subsystem4/2(CgXYZ)  "CgXYZ"
  AxlTrq/1 -> Longitudinal Wheels 4DOF/2(AxlTrq)
  Vehicle Body 3DOF External Longitudinal Wheels/1(" Info") -> Bus Selector13/1, Bus Selector11/1, Bus Selector10/1, Longitudinal Wheels 4DOF/6(VehFdbk), Bus Selector8/1, Bus Selector12/1, Bus Selector7/1, Bus Selector9/1, Bus Selector6/1, Bus Selector5/1
  [Ground] -> For 3D Visualization/3(GroundZ)
  Bus to Vector1/1 -> Subsystem4/3(CgXYZdot)  "CgXYZdot"
  Bus to Vector3/1 -> For 3D Visualization/1(angleIn)
  Longitudinal Wheels 4DOF/5(Alpha) -> Subsystem4/12(Alpha)  "Alpha"
  Vector Concatenate1/1 -> Longitudinal Wheels 4DOF/5(lam_mu), [mu]
  Bus Selector6/1 -> Bus to Vector1/1
  Brake Pressure/1(BrakePrs) -> Longitudinal Wheels 4DOF/3(BrkPrs)
  Vehicle Body 3DOF External Longitudinal Wheels/2(" XWheel") -> Subsystem4/13(XWheel)  "XWheel"
  Longitudinal Wheels 4DOF/4(Kappa) -> Subsystem4/11(Kappa)  "Kappa"
  Steering/1(WhlAng) -> Longitudinal Wheels 4DOF/1(WhlAng), Vehicle Body 3DOF External Longitudinal Wheels/1(WhlAng)
  Longitudinal Wheels 4DOF/6(zAxle) -> Subsystem4/15(dzWheel)  "dzWheel"
  Bus Selector7/1 -> Bus to Vector2/1
  Longitudinal Wheels 4DOF/3(Omega) -> Subsystem4/10(Omega)  "Omega"

== system EvBoltCalib_Lat_v1_comb/Vehicle/Vehicle Dynamics/Vehicle Longitudinal ==
  Env : Inport
  SupvsryCtrl : Inport  Port=2
  AxlTrq : Inport  Port=3
  Brake Pressure : Subsystem
  Bus Selector1 : BusSelector  OutputSignals=BrkCmd
  Bus Selector2 : BusSelector  OutputSignals=RoadGrade,WindVel,GndBus.z,GndBus.mu
  Bus Selector3 : BusSelector  OutputSignals=G_FL_z,G_FR_z,G_RL_z,G_RR_z
  Bus Selector4 : BusSelector  OutputSignals=mu_FL,mu_FR,mu_RL,mu_RR
  Constant : Constant  Value=0
  Longitudinal Wheels : Subsystem  AncestorBlock=LibWheels/Longitudinal Wheels and Brakes
      settings: LibrarySourceBlock=LibWheels/Longitudinal Wheels and Brakes
  Selector : Selector  InputPortWidth=3  IndexOptions=Index vector (dialog)  Indices=1  OutputSizes=1
  Terminator : Terminator
  Terminator1 : Terminator
  Vector Concatenate : Concatenate  NumInputs=4
  Vector Concatenate1 : Concatenate  NumInputs=4
  Vector Concatenate2 : Concatenate  NumInputs=4
  Vehicle Body : Subsystem
  Whl : Outport
  Chassis : Outport  Port=2
  wires:
  Vehicle Body/1(Chassis) -> Chassis/1
  Longitudinal Wheels/1(Whl) -> Whl/1
  Bus Selector4/1 -> Vector Concatenate1/1  "<mu_FL>"
  Bus Selector2/4 -> Bus Selector4/1  "<mu>"
  Vector Concatenate1/1 -> Terminator1/1
  Brake Pressure/1(BrakePrs) -> Longitudinal Wheels/1(BrkPrs)
  Bus Selector4/2 -> Vector Concatenate1/2  "<mu_FR>"
  Bus Selector3/1 -> Vector Concatenate/1  "<G_FL_z>"
  Bus Selector3/4 -> Vector Concatenate/4  "<G_RR_z>"
  Bus Selector2/3 -> Bus Selector3/1  "<z>"
  Env/1 -> Bus Selector2/1
  Vector Concatenate/1 -> Terminator/1
  Bus Selector4/3 -> Vector Concatenate1/3  "<mu_RL>"
  Bus Selector3/2 -> Vector Concatenate/2  "<G_FR_z>"
  SupvsryCtrl/1 -> Bus Selector1/1
  Constant/1 -> Vector Concatenate2/4, Vector Concatenate2/3, Vector Concatenate2/2, Vector Concatenate2/1
  Bus Selector4/4 -> Vector Concatenate1/4  "<mu_RR>"
  Bus Selector1/1 -> Brake Pressure/1(BrkReq)  "<BrkCmd>"
  Bus Selector3/3 -> Vector Concatenate/3  "<G_RL_z>"
  AxlTrq/1 -> Longitudinal Wheels/2(AxleTorq)
  Bus Selector2/2 -> Selector/1  "<WindVel>"
  Bus Selector2/1 -> Vehicle Body/1(RoadGrade)  "<RoadGrade>"
  Selector/1 -> Vehicle Body/2(WindX)
  connections:
  Longitudinal Wheels/RConn2 -- Vehicle Body/LConn2
  Vehicle Body/LConn1 -- Longitudinal Wheels/RConn1

== system EvBoltCalib_Lat_v1_comb/Vehicle/Battery/Battery/Lithium Ion Battery Pack1 ==
  note: Info
  BattCurr : Inport  Unit=A
  BattTemp : Inport  Port=2  Unit=K
  Datasheet Battery Internal : Subsystem  AncestorBlock=autolibbatterycommon/Datasheet Battery Internal
      settings: LibrarySourceBlock=autolibbatterycommon/Datasheet Battery Internal
  Info Bus : autolibbatterycommon/Info  RefBlkName='autolibdatasheetbattery/Datasheet Battery'
  Output Passthrough : autolibbatterycommon/Output Passthrough  SystemSampleTime=-1  VariantActivationTime=update diagram  Latency=0  AutoFrameSizeCalculation=off
  Info : Outport  VectorParamsAs1DForOutWhenUnconnected=off
  BattVolt : Outport  Port=2  Unit=V  VectorParamsAs1DForOutWhenUnconnected=off
  wires:
  [BattPwrLoss] -> Info Bus/5
  Output Passthrough/1 -> BattVolt/1, [BattVolt]
  [BattVolt] -> Info Bus/4
  Datasheet Battery Internal/1(LdCurrFeed) -> [LdCurrFeed]
  [LdCurrFeed] -> Info Bus/3
  Datasheet Battery Internal/5(BattPwrLoss) -> [BattPwrLoss]
  Datasheet Battery Internal/2(OutVoltUnfilt) -> Output Passthrough/1
  Datasheet Battery Internal/3(LdAmpHr) -> [LdAmpHr]
  Datasheet Battery Internal/4(BattSoc) -> [BattSoc]
  BattTemp/1 -> Datasheet Battery Internal/2(BattTemp)
  BattCurr/1 -> Datasheet Battery Internal/1(BattCurr)
  Info Bus/1 -> Info/1
  [BattSoc] -> Info Bus/2
  [LdAmpHr] -> Info Bus/1

== system EvBoltCalib_Lat_v1_comb/Vehicle/Front Wheel Drive/Ideal Diff/Power Bus ==
  DriveshftTrq : Inport
  Speed : Inport  Port=2
  Bus Creator : BusCreator  Inputs=1
  Bus Creator5 : BusCreator  Inputs=2
  Bus Creator6 : BusCreator  Inputs=3
  Bus Creator7 : BusCreator  Inputs=1
  Constant : Constant  Value=0
  Constant1 : Constant  Value=0
  Constant2 : Constant  Value=0
  Demux : Demux  Outputs=3
  Power Accounting Bus Creator : autolibpowerinfoutils/Power Accounting Bus Creator  AssctBlkSelPopup=Parent reference block  RefBlkName='autolibshareddiff/Open Differential'  PwrTrnsfrdCheckBox=on  PwrNotTrnsfrdCheckBox=on  PwrStoredCheckBox=on  aMode=aMode
  Signal Specification5 : SignalSpecification  Unit=W
  Transferred Power : Product
  Vector Concatenate : Concatenate  NumInputs=3
  PwrInfo : Outport
  wires:
  Bus Creator/1 -> Power Accounting Bus Creator/1
  Power Accounting Bus Creator/1 -> PwrInfo/1  "PwrInfo"
  Bus Creator5/1 -> Power Accounting Bus Creator/2
  Bus Creator6/1 -> Bus Creator/1  "PwrTrnsfrd"
  Transferred Power/1 -> Signal Specification5/1
  Signal Specification5/1 -> Vector Concatenate/3, Vector Concatenate/2, Vector Concatenate/1  "PwrDriveshft"
  Constant/1 -> Bus Creator5/1  "PwrMechLoss"
  Demux/3 -> Bus Creator6/3  "PwrAxl2"
  DriveshftTrq/1 -> Transferred Power/1
  Bus Creator7/1 -> Power Accounting Bus Creator/3
  Demux/2 -> Bus Creator6/2  "PwrAxl1"
  Demux/1 -> Bus Creator6/1  "PwrDriveshft"
  Speed/1 -> Transferred Power/2
  Vector Concatenate/1 -> Demux/1
  Constant1/1 -> Bus Creator5/2  "PwrDampLoss"
  Constant2/1 -> Bus Creator7/1  "PwrStoredShft"

== system EvBoltCalib_Lat_v1_comb/Vehicle/Front Wheel Drive/Real Diff/Power Bus ==
  DriveshftTrq : Inport
  Speed : Inport  Port=2
  Bus Creator : BusCreator  Inputs=1
  Bus Creator5 : BusCreator  Inputs=2
  Bus Creator6 : BusCreator  Inputs=3
  Bus Creator7 : BusCreator  Inputs=1
  Constant : Constant  Value=0
  Constant1 : Constant  Value=0
  Constant2 : Constant  Value=0
  Demux : Demux  Outputs=3
  Power Accounting Bus Creator : autolibpowerinfoutils/Power Accounting Bus Creator  AssctBlkSelPopup=Parent reference block  RefBlkName='autolibshareddiff/Open Differential'  PwrTrnsfrdCheckBox=on  PwrNotTrnsfrdCheckBox=on  PwrStoredCheckBox=on  aMode=aMode
  Signal Specification5 : SignalSpecification  Unit=W
  Transferred Power : Product
  Vector Concatenate : Concatenate  NumInputs=3
  PwrInfo : Outport
  wires:
  Bus Creator/1 -> Power Accounting Bus Creator/1
  Power Accounting Bus Creator/1 -> PwrInfo/1  "PwrInfo"
  Bus Creator5/1 -> Power Accounting Bus Creator/2
  Bus Creator6/1 -> Bus Creator/1  "PwrTrnsfrd"
  Transferred Power/1 -> Signal Specification5/1
  Signal Specification5/1 -> Vector Concatenate/3, Vector Concatenate/2, Vector Concatenate/1  "PwrDriveshft"
  Constant/1 -> Bus Creator5/1  "PwrMechLoss"
  Demux/3 -> Bus Creator6/3  "PwrAxl2"
  DriveshftTrq/1 -> Transferred Power/1
  Bus Creator7/1 -> Power Accounting Bus Creator/3
  Demux/2 -> Bus Creator6/2  "PwrAxl1"
  Demux/1 -> Bus Creator6/1  "PwrDriveshft"
  Speed/1 -> Transferred Power/2
  Vector Concatenate/1 -> Demux/1
  Constant1/1 -> Bus Creator5/2  "PwrDampLoss"
  Constant2/1 -> Bus Creator7/1  "PwrStoredShft"

== system EvBoltCalib_Lat_v1_comb/Vehicle/Powertrain Supervisory Controller /Engine Torque Command/Accel Pedal to Traction Wheel Torque Request1 ==
  note: Convert Accelerator Pedal Position to Torque Command
      | using Motor Torque Speed Curve
  AccelPdl : Inport
  MotSpd : Inport  Port=2
  Max Motor Torque : Subsystem
  Product1 : Product
  TrqCmd : Outport  VectorParamsAs1DForOutWhenUnconnected=off
  wires:
  Max Motor Torque/1(MtrTrqMax) -> Product1/2
  MotSpd/1 -> Max Motor Torque/1(MtrSpd)
  AccelPdl/1 -> Product1/1
  Product1/1 -> TrqCmd/1

== system EvBoltCalib_Lat_v1_comb/Vehicle/Powertrain Supervisory Controller /Engine Torque Command/Battery Management System ==
  note: Behaviorial BMS System. Limits battery charge / discharge power based on SOC.
      |
      | Charge/Discharge Limits and curves can be adjusted if using a larger battery pack
      | or motor power is changed.
  SOC : Inport
  ChrgLmt : Lookup_n-D  NumberOfTableDimensions=1  BreakpointsForDimension1=BattChargeLimitSocBpts  Table=BattChargeLimitTbl  ExtrapMethod=Clip  UseLastTableValue=on  InternalRulePriority=Speed  RndMeth=Simplest
  DischrgLmt : Lookup_n-D  NumberOfTableDimensions=1  BreakpointsForDimension1=BattDischargeLimitSocBpts  Table=BattDischargeLimitTbl  ExtrapMethod=Clip  UseLastTableValue=on  InternalRulePriority=Speed  RndMeth=Simplest
  MaxChrg : Constant  Value=BattChargeLimitMaxPwr
  MaxDischrg : Constant  Value=BattDischargeMaxPwr
  Product : Product
  Product1 : Product
  BattPwrDischrgLmt : Outport  VectorParamsAs1DForOutWhenUnconnected=off
  BattPwrChrgLmt : Outport  Port=2  VectorParamsAs1DForOutWhenUnconnected=off
  wires:
  DischrgLmt/1 -> Product/1
  ChrgLmt/1 -> Product1/1
  Product1/1 -> BattPwrChrgLmt/1
  Product/1 -> BattPwrDischrgLmt/1
  MaxDischrg/1 -> Product/2
  MaxChrg/1 -> Product1/2
  SOC/1 -> ChrgLmt/1, DischrgLmt/1

== system EvBoltCalib_Lat_v1_comb/Vehicle/Powertrain Supervisory Controller /Engine Torque Command/Motor Torque Arbitration and Power Management ==
  MotTrqCmdTrac : Inport
  AccelPdl : Inport  Port=2
  BattPwrDisChrgLmt : Inport  Port=3
  "BattPwrChrgLmt " : Inport  Port=4
  MotSpd : Inport  Port=5
  MotTrqCmdRegen : Inport  Port=6
  Accel Decel Switch : Switch  Criteria=u2 > Threshold  SaturateOnIntegerOverflow=off  InputSameDT=off
  Compare To Constant : simulink/Logic and Bit Operations/Compare To Constant  relop=>  const=0  OutDataTypeStr=boolean
  Power Management : Subsystem
  MotTrqCmdFinal : Outport  VectorParamsAs1DForOutWhenUnconnected=off
  wires:
  Compare To Constant/1 -> Accel Decel Switch/2
  MotSpd/1 -> Power Management/3(MotSpd)
  "BattPwrChrgLmt "/1 -> Power Management/2(BattPwrChrgLmt)
  BattPwrDisChrgLmt/1 -> Power Management/1(BattPwrDischrgLmt)
  Accel Decel Switch/1 -> Power Management/4(MotTrqCmd)
  Power Management/1(MotTrqCmdFinal) -> MotTrqCmdFinal/1
  MotTrqCmdTrac/1 -> Accel Decel Switch/1
  MotTrqCmdRegen/1 -> Accel Decel Switch/3
  AccelPdl/1 -> Compare To Constant/1
